simulink model "Simple_Pendulum_Motion_Simulation"  (R2019a)
settings: Solver=VariableStepAuto  StartTime=0.0  StopTime=10.0  MaxStep=0.001  RelTol=1e-3
undefined symbols (not defined in the file): g, L
settings Model: Creator=T.S  LastModifiedBy=T.S

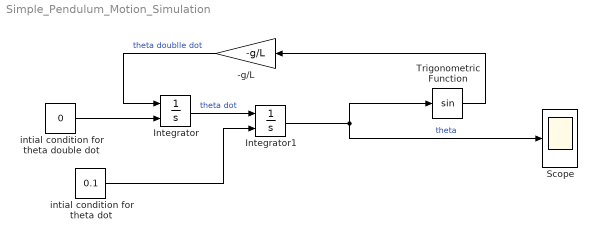
== system Simple_Pendulum_Motion_Simulation ==
  -g/L : Gain  Gain=-g/L
  Integrator : Integrator  InitialConditionSource=external
  Integrator1 : Integrator  InitialConditionSource=external
  Scope : Scope
  Trigonometric Function : Trigonometry
  intial condition for theta dot : Constant  Value=0.1
  intial condition for theta double dot : Constant  Value=0
  wires:
  Integrator1/1 -> Trigonometric Function/1, Scope/1  "theta"
  Integrator/1 -> Integrator1/1  "theta dot"
  Trigonometric Function/1 -> -g/L/1
  -g/L/1 -> Integrator/1  "theta doublle dot"
  intial condition for theta double dot/1 -> Integrator/2
  intial condition for theta dot/1 -> Integrator1/2
